simulink model "svpwm_modulator"  (R2023b)
settings: Solver=FixedStepDiscrete  StartTime=0.0  StopTime=0.01  FixedStep=Ts_mod  RelTol=1e-3
model workspace (MATLAB code in the model file):
  | % SVPWM modulator parameters
  | % Placeholder values for structural modelling only; no optimisation or hardware-timing detail intended.
  | 
  | Ts_mod = 1e-6;            % modulation discrete update period [s] (placeholder)
  | 
  | fsw = 5000;               % switching frequency [Hz] (placeholder)
libraries: simulink x1
settings Model: Creator=hwma  LastModifiedBy=hwma

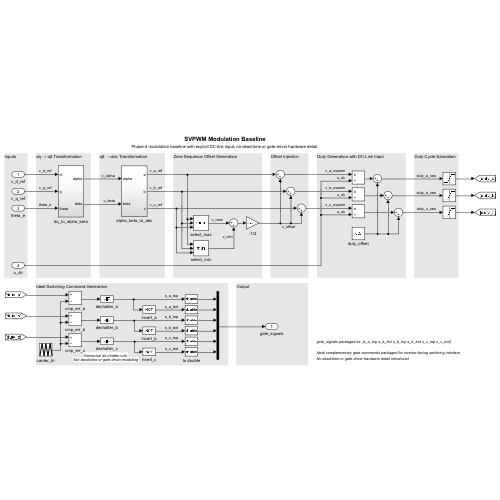
[thumbnail: Simulink's stored preview of the top-level diagram]
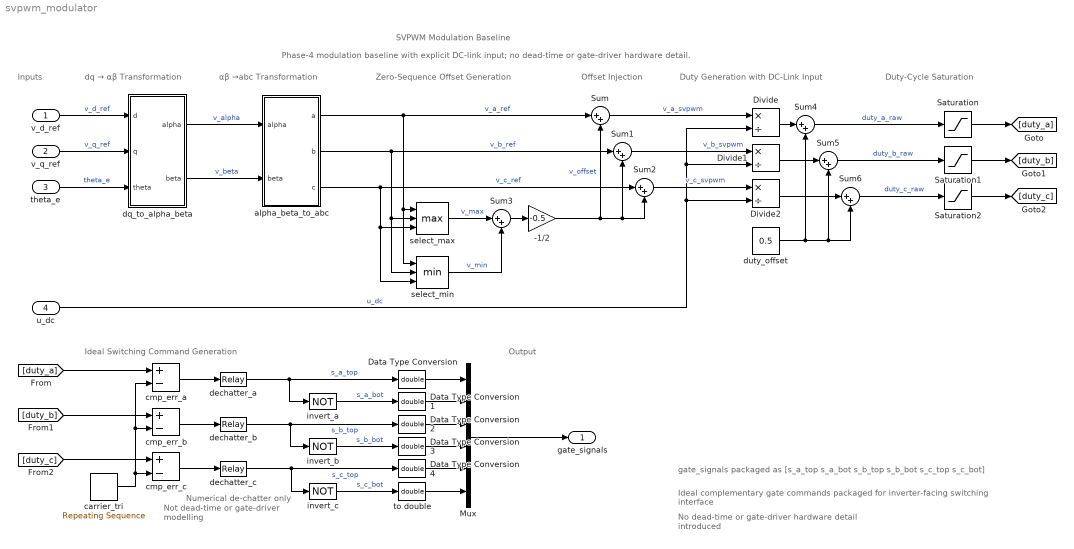
== system svpwm_modulator ==
  note: Ideal complementary gate commands packaged for inverter-facing switching interface
  note: gate_signals packaged as [s_a_top s_a_bot s_b_top s_b_bot s_c_top s_c_bot]
  note: Numerical de-chatter only
  note: Inputs
  note: SVPWM Modulation Baseline
  note: Phase-4 modulation baseline with explicit DC-link input; no dead-time or gate-driver hardware detail.
  note: dq → αβ Transformation
  note: αβ →abc Transformation
  note: Zero-Sequence Offset Generation
  note: Offset Injection
  note: Duty Generation with DC-Link Input
  note: Duty-Cycle Saturation
  note: Ideal Switching Command Generation
  note: Not dead-time or gate-driver modelling
  note: No dead-time or gate-driver hardware detail introduced
  note: Output
  v_d_ref : Inport
  v_q_ref : Inport  Port=2
  theta_e : Inport  Port=3
  u_dc : Inport  Port=4
  -1/2 : Gain  Gain=-0.5
  Data Type Conversion{,1..4} (5 alike) : DataTypeConversion  OutDataTypeStr=double  SaturateOnIntegerOverflow=off  RndMeth=Floor
  Divide : Product  Inputs=*/
  Divide1 : Product  Inputs=*/
  Divide2 : Product  Inputs=*/
  Mux : Mux  Inputs=6
  Saturation : Saturate  UpperLimit=1  LowerLimit=0
  Saturation1 : Saturate  UpperLimit=1  LowerLimit=0
  Saturation2 : Saturate  UpperLimit=1  LowerLimit=0
  Sum{,1..6} (7 alike) : Sum  Inputs=|++
  alpha_beta_to_abc : Subsystem
  carrier_tri : simulink/Sources/Repeating Sequence  rep_seq_t=[0 1/(2*fsw) 1/fsw]  rep_seq_y=[0 1 0]
  cmp_err_a : Sum  Inputs=+-
  cmp_err_b : Sum  Inputs=+-
  cmp_err_c : Sum  Inputs=+-
  dechatter_a : Relay  OnSwitchValue=1e-6  OffSwitchValue=-1e-6
  dechatter_b : Relay  OnSwitchValue=1e-6  OffSwitchValue=-1e-6
  dechatter_c : Relay  OnSwitchValue=1e-6  OffSwitchValue=-1e-6
  dq_to_alpha_beta : Subsystem
  duty_offset : Constant  Value=0.5
  invert_a : Logic  Operator=NOT  AllPortsSameDT=off  OutDataTypeStr=boolean
  invert_b : Logic  Operator=NOT  AllPortsSameDT=off  OutDataTypeStr=boolean
  invert_c : Logic  Operator=NOT  AllPortsSameDT=off  OutDataTypeStr=boolean
  select_max : MinMax  Function=max  Inputs=3
  select_min : MinMax  Inputs=3
  to double : DataTypeConversion  OutDataTypeStr=double  SaturateOnIntegerOverflow=off  RndMeth=Floor
  gate_signals : Outport
  wires:
  dq_to_alpha_beta/1(alpha) -> alpha_beta_to_abc/1(alpha)  "v_alpha"
  dq_to_alpha_beta/2(beta) -> alpha_beta_to_abc/2(beta)  "v_beta"
  alpha_beta_to_abc/2(b) -> Sum1/1, select_min/2, select_max/2  "v_b_ref"
  alpha_beta_to_abc/1(a) -> Sum/1, select_min/1, select_max/1  "v_a_ref"
  alpha_beta_to_abc/3(c) -> Sum2/1, select_max/3, select_min/3  "v_c_ref"
  select_max/1 -> Sum3/1  "v_max"
  select_min/1 -> Sum3/2  "v_min"
  Sum3/1 -> -1/2/1
  -1/2/1 -> Sum2/2, Sum1/2, Sum/2  "v_offset"
  Sum/1 -> Divide/1  "v_a_svpwm"
  Sum1/1 -> Divide1/1  "v_b_svpwm"
  Sum2/1 -> Divide2/1  "v_c_svpwm"
  Divide/1 -> Sum4/1
  Divide1/1 -> Sum5/1
  Divide2/1 -> Sum6/1
  duty_offset/1 -> Sum6/2, Sum5/2, Sum4/2
  Sum4/1 -> Saturation/1  "duty_a_raw"
  Sum5/1 -> Saturation1/1  "duty_b_raw"
  Sum6/1 -> Saturation2/1  "duty_c_raw"
  Saturation/1 -> [duty_a]
  Saturation1/1 -> [duty_b]
  Saturation2/1 -> [duty_c]
  [duty_a] -> cmp_err_a/1
  [duty_b] -> cmp_err_b/1
  [duty_c] -> cmp_err_c/1
  carrier_tri/1 -> cmp_err_c/2, cmp_err_b/2, cmp_err_a/2
  cmp_err_a/1 -> dechatter_a/1
  cmp_err_b/1 -> dechatter_b/1
  cmp_err_c/1 -> dechatter_c/1
  dechatter_a/1 -> Data Type Conversion/1, invert_a/1  "s_a_top"
  invert_a/1 -> Data Type Conversion1/1  "s_a_bot"
  invert_b/1 -> Data Type Conversion3/1  "s_b_bot"
  dechatter_b/1 -> invert_b/1, Data Type Conversion2/1  "s_b_top"
  dechatter_c/1 -> invert_c/1, Data Type Conversion4/1  "s_c_top"
  invert_c/1 -> to double/1  "s_c_bot"
  Data Type Conversion/1 -> Mux/1
  Data Type Conversion1/1 -> Mux/2
  Data Type Conversion2/1 -> Mux/3
  Data Type Conversion3/1 -> Mux/4
  Data Type Conversion4/1 -> Mux/5
  to double/1 -> Mux/6
  Mux/1 -> gate_signals/1
  v_d_ref/1 -> dq_to_alpha_beta/1(d)  "v_d_ref"
  v_q_ref/1 -> dq_to_alpha_beta/2(q)  "v_q_ref"
  theta_e/1 -> dq_to_alpha_beta/3(theta)  "theta_e"
  u_dc/1 -> Divide2/2, Divide1/2, Divide/2  "u_dc"

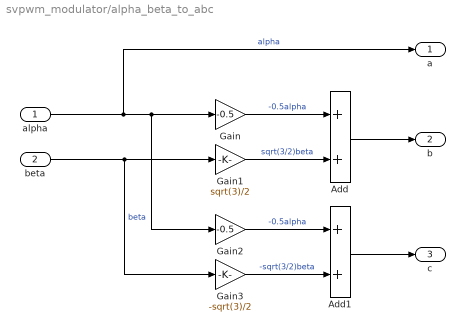
== system svpwm_modulator/alpha_beta_to_abc ==
  alpha : Inport
  beta : Inport  Port=2
  Add : Sum
  Add1 : Sum
  Gain : Gain  Gain=-0.5
  Gain1 : Gain  Gain=sqrt(3)/2
  Gain2 : Gain  Gain=-0.5
  Gain3 : Gain  Gain=-sqrt(3)/2
  a : Outport
  b : Outport  Port=2
  c : Outport  Port=3
  wires:
  beta/1 -> Gain1/1, Gain3/1  "beta"
  Add1/1 -> c/1
  alpha/1 -> a/1, Gain/1, Gain2/1  "alpha"
  Gain3/1 -> Add1/2  "-sqrt(3/2)beta"
  Gain1/1 -> Add/2  "sqrt(3/2)beta"
  Add/1 -> b/1
  Gain2/1 -> Add1/1  "-0.5alpha"
  Gain/1 -> Add/1  "-0.5alpha"

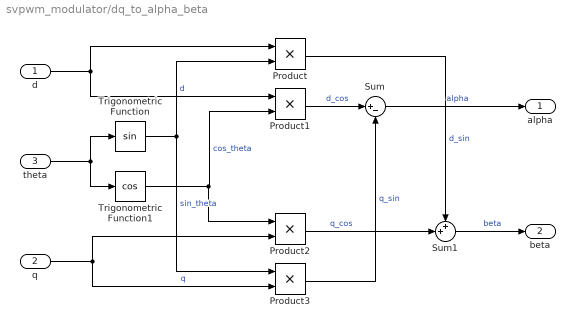
== system svpwm_modulator/dq_to_alpha_beta ==
  d : Inport
  q : Inport  Port=2
  theta : Inport  Port=3
  Product{,1..3} (4 alike) : Product
  Sum : Sum  Inputs=|+-
  Sum1 : Sum  Inputs=++|
  Trigonometric Function : Trigonometry
  Trigonometric Function1 : Trigonometry  Operator=cos
  alpha : Outport
  beta : Outport  Port=2
  wires:
  q/1 -> Product3/2, Product2/2  "q"
  Trigonometric Function1/1 -> Product2/1, Product1/2  "cos_theta"
  Product1/1 -> Sum/1  "d_cos"
  theta/1 -> Trigonometric Function/1, Trigonometric Function1/1
  Trigonometric Function/1 -> Product3/1, Product/2  "sin_theta"
  d/1 -> Product1/1, Product/1  "d"
  Product2/1 -> Sum1/2  "q_cos"
  Product3/1 -> Sum/2  "q_sin"
  Product/1 -> Sum1/1  "d_sin"
  Sum1/1 -> beta/1  "beta"
  Sum/1 -> alpha/1  "alpha"
